simulink model "actuator_2"  (R2020b)
settings: Solver=VariableStepAuto  StartTime=0.0  StopTime=50  FixedStep=0.01  MaxStep=0.1  RelTol=1e-3  AbsTol=1e-3  SampleTimeConstraint=STIndependent  EnableMultiTasking=on
PreLoadFcn:
  | % Pressure source
  | p_source = 8e5; % Pa
  | 
  | % 4-way directional valve
  | valve_area_max = 3e-5; % m^2
  | L0 = 1e-5;
  | 
  | % Pipes
  | L_pipe = 20; % m
  | flow_area = 1e-4; % m^2
  | 
  | % Air muscle actuators
  | L_muscle = 30; % cm
  | L_braid = 32; % cm
  | n = 2.5;
  | 
  | % Flow control valves
  | dp_crack = 1e4; % Pa
  | dp_max = 2e4; % Pa
  | area_max = 1e-5; % m^2
  | area_leak = 1e-10; % m^2
  | area_restrict = 1e-6; % m^2
  | 
  | % Translational dampers
  | D_translation = 1; % N/(m/s)
  | 
  | % Translational hard stops
  | x_bound = 8; % cm
  | 
  | % Linkage
  | L_top = 15; % cm
  | L_bottom = 15; % cm
  | 
  | % Load
  | inertia = 0.005; % kg*m^2
  | D_rotation = 10; % N*m/(rad/s)
  | K_spring = 6.4; % N*m/rad
  | theta_upper = 0.4; % rad
  | theta_lower = 0; % rad
  | 
  | % Environment
  | T_atm = 293.15; % K
  | p_atm = 0.101325; % MPa
InitFcn:
  | set_param('actuator_2','SimulationCommand','pause');
StartFcn:
  | set_param('actuator_2','SimulationCommand','pause');
libraries: fl_lib x26, SimscapeFluids_lib x8, fl_ps_legacy_lib x8, nesl_utility x7, dsparch4 x2, pid_lib x2
(part 1 of 3)
CloseFcn:
  | try,close(h1_sscfluids_antagonistic_mckibben_actuator),end
  | clear h1_sscfluids_antagonistic_mckibben_actuator
  | try,close(h2_sscfluids_antagonistic_mckibben_actuator),end
  | clear h2_sscfluids_antagonistic_mckibben_actuator
  | 
  | clear simlog_sscfluids_antagonistic_mckibben_actuator tout
  | clear T_atm p_atm p_source flow_area
  | clear valve_area_max L0 L_pipe dp_crack dp_max
  | clear area_max area_leak area_restrict
  | clear L_muscle L_braid n D_translation x_bound
  | clear L_top L_bottom inertia D_rotation K_spring
  | clear theta_upper theta_lower
Description:
  | Antagonistic McKibben Muscle Actuator
settings Model: Tag=PublishSubsystemCustomStyle  PacingRate=10  Creator=The MathWorks, Inc.  LastModifiedBy=zhb
settings SolverCC: AutoScaleAbsTol=off
settings DataIOCC: MaxDataPoints=10000  SignalLogging=off  ReturnWorkspaceOutputs=off  SignalLoggingName=logsout_sscfluids_antagonistic_mckibben_actuator
settings OptimizationCC: LifeSpan=inf
settings DebuggingCC: AllowSymbolicDim=off  PregeneratedLibrarySubsystemCodeDiagnostic=none  SFUnexpectedBacktrackingDiag=warning  SFNoUnconditionalDefaultTransitionDiag=warning  SFExecutionAtInitializationDiag=none  ArithmeticOperatorsInVariantConditions=warning
settings SFSimCC: SimUseLocalCustomCode=off  CustomCodeUndefinedFunction=UseInterfaceOnly
settings RTWCC: RTWUseLocalCustomCode=off
settings CodeAppCC: StateflowObjectComments=on
settings GRTTargetCC: TargetLangStandard=C89/C90 (ANSI)
settings ConfigComp: CovMetricSettings=dw  CovSaveCumulativeToWorkspaceVar=on  CovSaveSingleToWorkspaceVar=on  CovExternalEMLEnable=off  CovSFcnEnable=off
settings SimscapeCC: SimscapeLogType=all  SimscapeLogSimulationStatistics=on  SimscapeLogName=simlog_sscfluids_antagonistic_mckibben_actuator  SimscapeLogLimitData=off  SimscapeLogDataHistory=10000

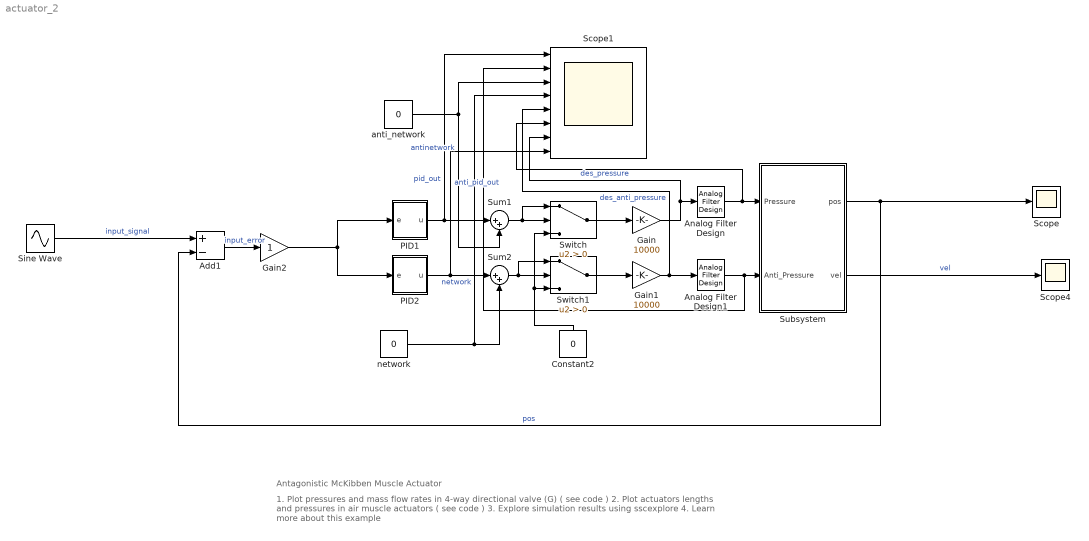
== system actuator_2 ==
  note: Antagonistic McKibben Muscle Actuator
  note: 1. Plot pressures and mass flow rates in 4-way directional valve (G) ( see code )
      | 2. Plot actuators lengths and pressures in air muscle actuators ( see code )
      | 3. Explore simulation results using sscexplore
      | 4. Learn more about this example
  Add1 : Sum  Inputs=+-
  Analog Filter Design : dsparch4/Analog Filter Design  method=Butterworth  filttype=Lowpass  N=8  Wlo=30  Whi=80  Rp=2  Rs=40
  Analog Filter Design1 : dsparch4/Analog Filter Design  method=Butterworth  filttype=Lowpass  N=8  Wlo=30  Whi=80  Rp=2  Rs=40
  Constant2 : Constant  Value=0
  Gain : Gain  Gain=10000
  Gain1 : Gain  Gain=10000
  Gain2 : Gain
  PID1 : Subsystem  mask{Kc=-0.7500, Td=0.0, Ti=30.0, Ad=10, U0=0}
      mask Display: disp('PID(s)')
  PID2 : Subsystem  mask{Kc=0.75, Td=0.0, Ti=30.0, Ad=10, U0=0}
      mask Display: disp('PID(s)')
  Scope : Scope
  Scope1 : Scope  NumInputPorts=8
  Scope4 : Scope
  Sine Wave : Sin  Amplitude=2.4  Bias=2.4  Frequency=0.2  Phase=-pi/2  SampleTime=0
  Subsystem : Subsystem
  Sum1 : Sum  Inputs=|++
  Sum2 : Sum  Inputs=|++
  Switch : Switch  Criteria=u2 > Threshold
  Switch1 : Switch  Criteria=u2 > Threshold
  anti_network : Constant  Value=0
  network : Constant  Value=0
  wires:
  PID1/1("u ") -> Scope1/1, Sum1/1  "pid_out"
  Sine Wave/1 -> Add1/1  "input_signal"
  Subsystem/1(pos) -> Scope/1, Add1/2  "pos"
  PID2/1("u ") -> Scope1/8, Sum2/1  "anti_pid_out"
  Subsystem/2(vel) -> Scope4/1  "vel"
  network/1 -> Sum2/2, Scope1/4  "network"
  Gain/1 -> Analog Filter Design/1, Scope1/7  "des_pressure"
  Gain1/1 -> Analog Filter Design1/1, Scope1/5  "des_anti_pressure"
  Sum1/1 -> Switch/1, Switch/2
  Switch/1 -> Gain/1
  Switch1/1 -> Gain1/1
  Sum2/1 -> Switch1/1, Switch1/2
  Constant2/1 -> Switch1/3, Switch/3
  anti_network/1 -> Scope1/3, Sum1/2  "antinetwork"
  Add1/1 -> Gain2/1  "input_error"
  Gain2/1 -> PID2/1(e), PID1/1(e)
  Analog Filter Design/1 -> Scope1/6, Subsystem/1(Pressure)
  Analog Filter Design1/1 -> Scope1/2, Subsystem/2(Anti_Pressure)

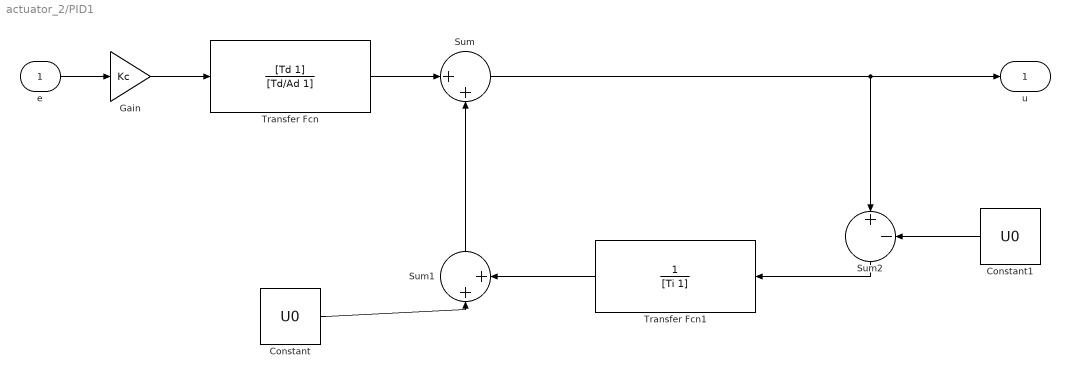
== system actuator_2/PID1 ==
  e : Inport
  Constant : Constant  Value=U0
  Constant1 : Constant  Value=U0
  Gain : Gain  Gain=Kc
  Sum : Sum  Inputs=|++
  Sum1 : Sum  Inputs=|++
  Sum2 : Sum  Inputs=|+-
  Transfer Fcn : TransferFcn  Numerator=[Td 1]  Denominator=[Td/Ad 1]
  Transfer Fcn1 : TransferFcn  Denominator=[Ti 1]
  "u " : Outport  VectorParamsAs1DForOutWhenUnconnected=off
  wires:
  e/1 -> Gain/1
  Constant/1 -> Sum1/1
  Gain/1 -> Transfer Fcn/1
  Transfer Fcn1/1 -> Sum1/2
  Transfer Fcn/1 -> Sum/1
  Sum1/1 -> Sum/2
  Constant1/1 -> Sum2/2
  Sum2/1 -> Transfer Fcn1/1
  Sum/1 -> Sum2/1, "u "/1

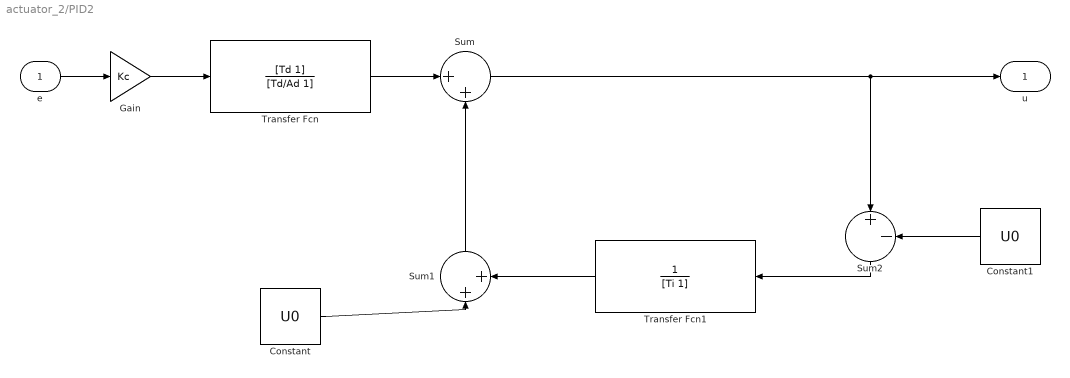
== system actuator_2/PID2 ==
  e : Inport
  Constant : Constant  Value=U0
  Constant1 : Constant  Value=U0
  Gain : Gain  Gain=Kc
  Sum : Sum  Inputs=|++
  Sum1 : Sum  Inputs=|++
  Sum2 : Sum  Inputs=|+-
  Transfer Fcn : TransferFcn  Numerator=[Td 1]  Denominator=[Td/Ad 1]
  Transfer Fcn1 : TransferFcn  Denominator=[Ti 1]
  "u " : Outport  VectorParamsAs1DForOutWhenUnconnected=off
  wires:
  e/1 -> Gain/1
  Constant/1 -> Sum1/1
  Gain/1 -> Transfer Fcn/1
  Transfer Fcn1/1 -> Sum1/2
  Transfer Fcn/1 -> Sum/1
  Sum1/1 -> Sum/2
  Constant1/1 -> Sum2/2
  Sum2/1 -> Transfer Fcn1/1
  Sum/1 -> "u "/1, Sum2/1
